simulink model "abs_EV_SLC"  (R2023a)
settings: Solver=ode45  StartTime=0  StopTime=15  FixedStep=0.002  RelTol=1e-3  AbsTol=1e-6
libraries: cstblocks x2, simulink x2, Solver_SF x1
settings Model: ExtModeTrigMode=oneshot  VariantFading=off  Creator=ywata  LastModifiedBy=USER
settings SolverCC: AutoScaleAbsTol=off  AlgebraicLoopSolver=TrustRegion
settings DataIOCC: SaveFormat=Array  SignalLoggingSaveFormat=ModelDataLogs  ReturnWorkspaceOutputs=off  SignalLoggingName=sigsOut
settings OptimizationCC: BlockReduction=off  BooleanDataType=off  ExpressionDepthLimit=2147483647  LifeSpan=inf
settings DebuggingCC: SaveWithParameterizedLinksMsg=none  UnderspecifiedInitializationDetection=Classic  MergeDetectMultiDrivingBlocksExec=none  SignalResolutionControl=TryResolveAllWithWarning  MultiTaskDSMMsg=warning  MultiTaskCondExecSysMsg=none  FcnCallInpInsideContextMsg=warning  UnconnectedInputMsg=warning  UnconnectedOutputMsg=warning  UnconnectedLineMsg=warning  StateNameClashWarn=warning  SFUnexpectedBacktrackingDiag=warning  SFNoUnconditionalDefaultTransitionDiag=warning  SFExecutionAtInitializationDiag=none  ArithmeticOperatorsInVariantConditions=warning
settings HardwareCC: ProdBitPerPointer=32  ProdBitPerSizeT=32  ProdBitPerPtrDiffT=32  ProdLargestAtomicFloat=None  ProdIntDivRoundTo=Undefined  ProdEndianess=Unspecified  ProdWordSize=32  ProdHWDeviceType=32-bit Generic  TargetUnknown=on
settings ModelReferenceCC: PropagateSignalLabelsOutOfModel=off
settings SFSimCC: SimUseLocalCustomCode=off  CustomCodeUndefinedFunction=UseInterfaceOnly
settings RTWCC: TemplateMakefile=grt_vc.tmf  RTWUseLocalCustomCode=off
settings CodeAppCC: StateflowObjectComments=on
settings GRTTargetCC: TargetFcnLib=ansi_tfl_tmw.mat  TargetLangStandard=C89/C90 (ANSI)  CombineOutputUpdateFcns=off  GRTInterface=on
settings ConfigComp: CovMetricSettings=dw  CovSaveCumulativeToWorkspaceVar=on  CovSaveSingleToWorkspaceVar=on  CovExternalEMLEnable=off

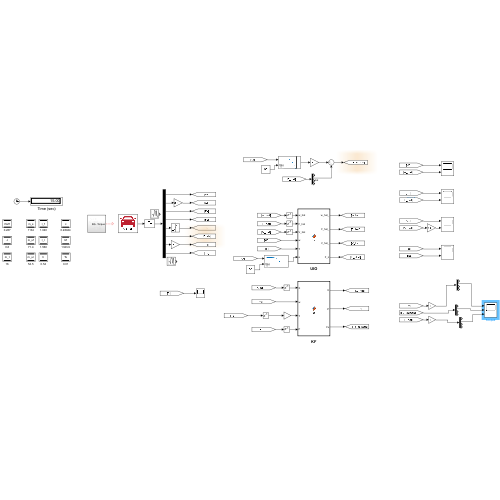
[thumbnail: Simulink's stored preview of the top-level diagram]
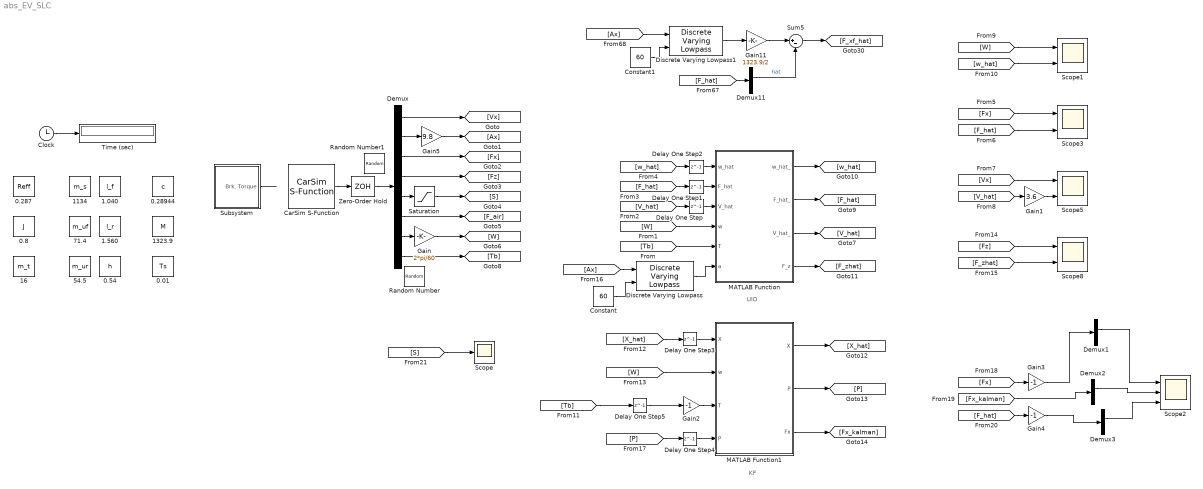
== system abs_EV_SLC ==
  note: UIO
  note: KF
  0.01 : DataStoreMemory  DataStoreName=Ts  WriteAfterWriteMsg=warning  InitialValue=0.01  ShowAdditionalParam=off  OutDataTypeStr=double
  0.287 : DataStoreMemory  DataStoreName=Reff  WriteAfterWriteMsg=warning  InitialValue=0.287  ShowAdditionalParam=off  OutDataTypeStr=double
  0.28944 : DataStoreMemory  DataStoreName=c  WriteAfterWriteMsg=warning  InitialValue=0.29844  ShowAdditionalParam=off  OutDataTypeStr=double
  0.54 : DataStoreMemory  DataStoreName=h  WriteAfterWriteMsg=warning  InitialValue=0.54  ShowAdditionalParam=off  OutDataTypeStr=double
  0.8 : DataStoreMemory  DataStoreName=J  WriteAfterWriteMsg=warning  InitialValue=0.8  ShowAdditionalParam=off  OutDataTypeStr=double
  1.040 : DataStoreMemory  DataStoreName=l_f  WriteAfterWriteMsg=warning  InitialValue=1.040  ShowAdditionalParam=off  OutDataTypeStr=double
  1.560 : DataStoreMemory  DataStoreName=l_r  WriteAfterWriteMsg=warning  InitialValue=1.560  ShowAdditionalParam=off  OutDataTypeStr=double
  1134 : DataStoreMemory  DataStoreName=m_s  WriteAfterWriteMsg=warning  InitialValue=1134  ShowAdditionalParam=off  OutDataTypeStr=double
  1323.9 : DataStoreMemory  DataStoreName=M  WriteAfterWriteMsg=warning  InitialValue=1323.9  ShowAdditionalParam=off  OutDataTypeStr=double
  16 : DataStoreMemory  DataStoreName=m_t  WriteAfterWriteMsg=warning  InitialValue=16  ShowAdditionalParam=off  OutDataTypeStr=double
  54.5 : DataStoreMemory  DataStoreName=m_ur  WriteAfterWriteMsg=warning  InitialValue=54.5  ShowAdditionalParam=off  OutDataTypeStr=double
  71.4 : DataStoreMemory  DataStoreName=m_uf  WriteAfterWriteMsg=warning  InitialValue=71.4  ShowAdditionalParam=off  OutDataTypeStr=double
  CarSim S-Function : Solver_SF/CarSim S-Function  Priority=1  SIMFILE=simfile.sim  Run_RTs=off  vs_state_ind=Run  StopMode_ind=Vehicle Model
  Clock : Clock
  Constant : Constant  Value=60
  Constant1 : Constant  Value=60
  Delay One Step : Delay  DelayLength=1  InitialCondition=19.444
  Delay One Step1 : Delay  DelayLength=1  InitialCondition=[0 0 0 0]'
  Delay One Step2 : Delay  DelayLength=1  InitialCondition=[67.655 67.655 67.655 67.655]'
  Delay One Step3 : Delay  DelayLength=1  InitialCondition=[67.655 67.655 67.655 67.655; 0 0 0 0]
  Delay One Step4 : Delay  DelayLength=1  InitialCondition=10*ones(2,8)
  Delay One Step5 : Delay  DelayLength=1  InitialCondition=[0 0 0 0]'
  Demux : Demux  Outputs=[1 1 4 4 4 1 4 4]
  Demux{1..3,11} (4 alike) : Demux
  Discrete Varying Lowpass : cstblocks/Linear Parameter Varying/Discrete Varying Lowpass  N=1  w0=0  Ts=0.01
  Discrete Varying Lowpass1 : cstblocks/Linear Parameter Varying/Discrete Varying Lowpass  N=1  w0=0  Ts=0.01
  Gain : Gain  Gain=2*pi/60
  Gain1 : Gain  Gain=3.6
  Gain11 : Gain  Gain=1323.9/2
  Gain2 : Gain  Gain=-1
  Gain3 : Gain  Gain=-1
  Gain4 : Gain  Gain=-1
  Gain5 : Gain  Gain=9.8
  MATLAB Function : MATLAB Function  TreatAsAtomicUnit=on
  MATLAB Function1 : MATLAB Function  TreatAsAtomicUnit=on
  Random Number : RandomNumber  Variance=0.01^2  SampleTime=0.01
  Random Number1 : RandomNumber  Variance=0.01  SampleTime=0.01
  Saturation : Saturate  UpperLimit=1  LowerLimit=-1
  Scope : Scope
  Scope{1,3,5,8} (4 alike) : Scope  NumInputPorts=2
  Scope2 : Scope  NumInputPorts=3
  Subsystem : Subsystem
  Sum5 : Sum  Inputs=|+-
  Time (sec) : Display
      settings: Format=bank  Decimation=100
  Zero-Order Hold : ZeroOrderHold  SampleTime=0.01
  wires:
  CarSim S-Function/1 -> Zero-Order Hold/1
  Clock/1 -> Time (sec)/1
  Demux/1 -> [Vx]
  Demux/3 -> [Fx]
  Demux/4 -> [Fz]
  Demux/7 -> Gain/1
  Demux/8 -> [Tb]
  Zero-Order Hold/1 -> Demux/1
  [Tb] -> MATLAB Function/5(T)
  [W] -> MATLAB Function/4(w)
  MATLAB Function/3(V_hat_) -> [V_hat]
  MATLAB Function/2(F_hat_) -> [F_hat]
  MATLAB Function/1(w_hat_) -> [w_hat]
  [V_hat] -> Delay One Step/1
  Delay One Step/1 -> MATLAB Function/3(V_hat)
  [F_hat] -> Delay One Step1/1
  Delay One Step1/1 -> MATLAB Function/2(F_hat)
  [w_hat] -> Delay One Step2/1
  Delay One Step2/1 -> MATLAB Function/1(w_hat)
  [Fx] -> Scope3/1
  [F_hat] -> Scope3/2
  [V_hat] -> Gain1/1
  [Vx] -> Scope5/1
  Gain1/1 -> Scope5/2
  [W] -> Scope1/1
  [w_hat] -> Scope1/2
  Demux/6 -> [F_air]
  MATLAB Function/4(F_z) -> [F_zhat]
  [F_zhat] -> Scope8/2
  [Fz] -> Scope8/1
  [Ax] -> Discrete Varying Lowpass/1
  Demux/5 -> Saturation/1
  Saturation/1 -> [S]
  [F_hat] -> Demux11/1
  Demux11/2 -> Sum5/2  "hat"
  [Ax] -> Discrete Varying Lowpass1/1
  Gain11/1 -> Sum5/1
  Sum5/1 -> [F_xf_hat]
  Gain/1 -> [W]
  Demux/2 -> Gain5/1
  Constant/1 -> Discrete Varying Lowpass/2
  Discrete Varying Lowpass/1 -> MATLAB Function/6(a)
  Gain5/1 -> [Ax]
  Constant1/1 -> Discrete Varying Lowpass1/2
  Discrete Varying Lowpass1/1 -> Gain11/1
  Subsystem/1(Brk. Torque) -> ?
  [Tb] -> Delay One Step5/1
  Gain2/1 -> MATLAB Function1/3(T)
  MATLAB Function1/1(X) -> [X_hat]
  [X_hat] -> Delay One Step3/1
  Delay One Step3/1 -> MATLAB Function1/1("X ")
  [W] -> MATLAB Function1/2(w)
  [P] -> Delay One Step4/1
  Delay One Step4/1 -> MATLAB Function1/4("P ")
  MATLAB Function1/2(P) -> [P]
  MATLAB Function1/3(Fx) -> [Fx_kalman]
  [Fx] -> Gain3/1
  [Fx_kalman] -> Demux2/1
  Gain3/1 -> Demux1/1
  [F_hat] -> Gain4/1
  Gain4/1 -> Demux3/1
  [S] -> Scope/1
  Demux1/2 -> Scope2/1
  Demux2/2 -> Scope2/2
  Demux3/2 -> Scope2/3
  Delay One Step5/1 -> Gain2/1

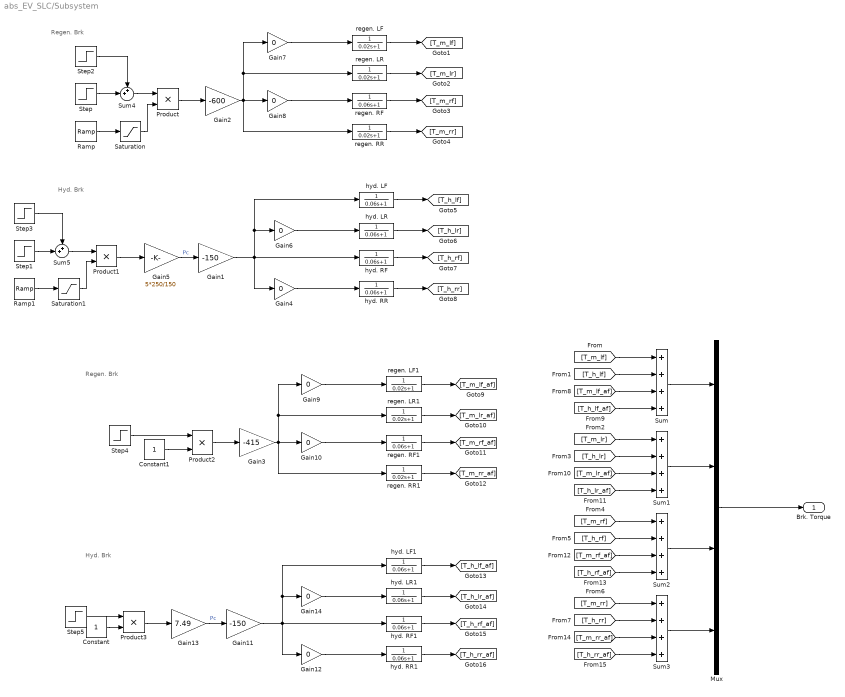
== system abs_EV_SLC/Subsystem ==
  note: Regen. Brk
  note: Hyd. Brk
  note: Regen. Brk
  note: Hyd. Brk
  Constant : Constant
  Constant1 : Constant
  Gain1 : Gain  Gain=-150
  Gain{4,6..10,12,14} (8 alike) : Gain  Gain=0
  Gain11 : Gain  Gain=-150
  Gain13 : Gain  Gain=7.49
  Gain2 : Gain  Gain=-600
  Gain3 : Gain  Gain=-415
  Gain5 : Gain  Gain=5*250/150
  Mux : Mux
  Product{,1..3} (4 alike) : Product
  Ramp : simulink/Sources/Ramp  slope=1/0.3  start=3  InitialOutput=0
  Ramp1 : simulink/Sources/Ramp  slope=1/0.3  start=3  InitialOutput=0
  Saturation : Saturate  UpperLimit=1  LowerLimit=0
  Saturation1 : Saturate  UpperLimit=1  LowerLimit=0
  Step : Step  Time=3  SampleTime=0.01
  Step1 : Step  Time=3  SampleTime=0.01
  Step2 : Step  Time=3.32  After=-1  SampleTime=0.01
  Step3 : Step  Time=3.32  After=-1  SampleTime=0.01
  Step4 : Step  Time=3.32  SampleTime=0.01
  Step5 : Step  Time=3.32  SampleTime=0.01
  Sum{,1..3} (4 alike) : Sum  Inputs=++++
  Sum4 : Sum  Inputs=++|
  Sum5 : Sum  Inputs=++|
  hyd. LF : TransferFcn  Denominator=[0.06 1]
  hyd. LF1 : TransferFcn  Denominator=[0.06 1]
  hyd. LR : TransferFcn  Denominator=[0.06 1]
  hyd. LR1 : TransferFcn  Denominator=[0.06 1]
  hyd. RF : TransferFcn  Denominator=[0.06 1]
  hyd. RF1 : TransferFcn  Denominator=[0.06 1]
  hyd. RR : TransferFcn  Denominator=[0.06 1]
  hyd. RR1 : TransferFcn  Denominator=[0.06 1]
  regen. LF : TransferFcn  Denominator=[0.02 1]
  regen. LF1 : TransferFcn  Denominator=[0.02 1]
  regen. LR : TransferFcn  Denominator=[0.02 1]
  regen. LR1 : TransferFcn  Denominator=[0.02 1]
  regen. RF : TransferFcn  Denominator=[0.06 1]
  regen. RF1 : TransferFcn  Denominator=[0.06 1]
  regen. RR : TransferFcn  Denominator=[0.02 1]
  regen. RR1 : TransferFcn  Denominator=[0.02 1]
  Brk. Torque : Outport
  wires:
  Saturation/1 -> Product/2
  Product/1 -> Gain2/1
  Ramp/1 -> Saturation/1
  Gain2/1 -> regen. RR/1, regen. LR/1, Gain7/1, Gain8/1
  regen. LF/1 -> [T_m_lf]
  regen. LR/1 -> [T_m_lr]
  regen. RF/1 -> [T_m_rf]
  regen. RR/1 -> [T_m_rr]
  Ramp1/1 -> Saturation1/1
  Product1/1 -> Gain5/1
  Saturation1/1 -> Product1/2
  hyd. RF/1 -> [T_h_rf]
  hyd. RR/1 -> [T_h_rr]
  hyd. LR/1 -> [T_h_lr]
  Gain6/1 -> hyd. LR/1
  Gain4/1 -> hyd. RR/1
  hyd. LF/1 -> [T_h_lf]
  Sum/1 -> Mux/1
  [T_m_lf] -> Sum/1
  [T_h_lf] -> Sum/2
  Mux/1 -> Brk. Torque/1
  Gain7/1 -> regen. LF/1
  Gain8/1 -> regen. RF/1
  Gain1/1 -> hyd. RF/1, hyd. LF/1, Gain6/1, Gain4/1
  Gain5/1 -> Gain1/1  "Pc"
  Step/1 -> Sum4/2
  Sum4/1 -> Product/1
  Step2/1 -> Sum4/1
  Step3/1 -> Sum5/1
  Step1/1 -> Sum5/2
  Sum5/1 -> Product1/1
  Step4/1 -> Product2/1
  Gain10/1 -> regen. RF1/1
  Gain3/1 -> regen. RR1/1, regen. LR1/1, Gain9/1, Gain10/1
  regen. LR1/1 -> [T_m_lr_af]
  regen. RF1/1 -> [T_m_rf_af]
  regen. LF1/1 -> [T_m_lf_af]
  Gain9/1 -> regen. LF1/1
  Product2/1 -> Gain3/1
  regen. RR1/1 -> [T_m_rr_af]
  Gain13/1 -> Gain11/1  "Pc"
  Gain11/1 -> hyd. RF1/1, hyd. LF1/1, Gain14/1, Gain12/1
  hyd. LF1/1 -> [T_h_lf_af]
  Gain12/1 -> hyd. RR1/1
  Product3/1 -> Gain13/1
  hyd. LR1/1 -> [T_h_lr_af]
  hyd. RF1/1 -> [T_h_rf_af]
  hyd. RR1/1 -> [T_h_rr_af]
  Gain14/1 -> hyd. LR1/1
  Step5/1 -> Product3/1
  [T_m_lf_af] -> Sum/3
  [T_h_lf_af] -> Sum/4
  [T_m_lr_af] -> Sum1/3
  [T_m_lr] -> Sum1/1
  [T_h_lr_af] -> Sum1/4
  [T_h_lr] -> Sum1/2
  Sum1/1 -> Mux/2
  [T_m_rf_af] -> Sum2/3
  [T_m_rf] -> Sum2/1
  [T_h_rf_af] -> Sum2/4
  [T_h_rf] -> Sum2/2
  Sum2/1 -> Mux/3
  [T_m_rr_af] -> Sum3/3
  [T_m_rr] -> Sum3/1
  [T_h_rr_af] -> Sum3/4
  [T_h_rr] -> Sum3/2
  Sum3/1 -> Mux/4
  Constant/1 -> Product3/2
  Constant1/1 -> Product2/2

== matlab function abs_EV_SLC/MATLAB Function1 ==
  data: X input; w input; T input; X output; P output; P input; Fx output; c data_store_memory; Reff data_store_memory; J data_store_memory; M data_store_memory; Ts data_store_memory; m_s data_store_memory; m_uf data_store_memory; m_ur data_store_memory; m_t data_store_memory; l_f data_store_memory; l_r data_store_memory; h data_store_memory
function [X,P,Fx]  = fcn(X,w,T,P)

global  Reff J Ts;

Qlf = [1 0;0 500000]; Qlr = [0.01 0;0 900]; Qrf = [1 0;0 500000]; Qrr = [1 0;0 500000]; Q = [Qlf Qlr Qrf Qrr];
Rlf = 1; Rlr = 0.01; Rrf = 1; Rrr = 1; R = [Rlf Rlr Rrf Rrr];

F = [1 Reff/J*Ts;0 1]; G = [-1/J*Ts;0]; H = [1 0];

for i = 1:4
    xm = F*X(:,i)+G*T(i);
    Pm = F*P(:,2*i-1:2*i)*F'+Q(:,2*i-1:2*i);
    K = Pm*H'/(H*Pm*H'+R(i));
    X(:,i) = xm+K*(w(i)-H*xm);
    P(:,2*i-1:2*i) = (eye(2)-K*H)*Pm;
end
Fx = X(2,:);

== matlab function abs_EV_SLC/MATLAB Function ==
  data: w_hat input; w_hat_ output; F_hat input; V_hat input; w input; T input; F_hat_ output; V_hat_ output; c data_store_memory; Reff data_store_memory; J data_store_memory; M data_store_memory; Ts data_store_memory; m_s data_store_memory; m_uf data_store_memory; m_ur data_store_memory; m_t data_store_memory; l_f data_store_memory; l_r data_store_memory; h data_store_memory; F_z output; a input
function [w_hat_,F_hat_,V_hat_,F_z]  = fcn(w_hat,F_hat,V_hat,w,T,a)

global c Reff J M Ts m_s m_uf m_ur m_t l_f l_r h;
l1 = 100; l2 = -8000;
X = [w_hat(1),F_hat(1),w_hat(2),F_hat(2),w_hat(3),F_hat(3),w_hat(4),F_hat(4),V_hat]';
U = [T(1)/J,0,T(2)/J,0,T(3)/J,0,T(4)/J,0,-c/M*V_hat^2]';
Y = [w(1), 0, w(2), 0, w(3), 0, w(4), 0, 0]';

A = [0 -Reff/J zeros(1,7); zeros(1,9); zeros(1,2) 0 -Reff/J zeros(1,5); zeros(1,9); zeros(1,4) 0 -Reff/J zeros(1,3); zeros(1,9); zeros(1,6) 0 -Reff/J 0; zeros(1,9); 0 1/M 0 1/M 0 1/M 0 1/M 0];
B = eye(9);
C = [1 0 zeros(1,7); zeros(1,9); zeros(1,2) 1 0 zeros(1,5); zeros(1,9); zeros(1,4) 1 0 zeros(1,3); zeros(1,9); zeros(1,6) 1 0 zeros(1,1); zeros(1,9); zeros(1,9);];
L0 = [l1 0;l2 0]; L = [L0 zeros(2,7); zeros(2,2) L0 zeros(2,5); zeros(2,4) L0 zeros(2,3); zeros(2,6) L0 zeros(2,1); zeros(1,9)];
X_ = (eye(9)+A*Ts)*X + Ts*B*U + Ts*L*(Y-C*X);

w_hat_ = X_([1,3,5,7]); F_hat_ = X_([2,4,6,8]); V_hat_ = X_(9);

%Fz
F_zf = ((m_s*l_r + (m_uf + 2*m_t)*(l_f + l_r))*9.8 - m_s*h*a)/(2*(l_f+l_r));
F_zr = ((m_s*l_f + (m_ur + 2*m_t)*(l_f + l_r))*9.8 + m_s*h*a)/(2*(l_f+l_r));

F_z = [F_zf F_zr F_zf F_zr]';
end
